simulink model "Modell_13_1"  (R2018a)
settings: Solver=VariableStepAuto  StartTime=0.0  StopTime=10.0  RelTol=1e-3
InitFcn:
  | init_13_1
values from neighbouring files (symbols this model uses):
  b = 1    [init_13_1.m]    (also in init_13_3.m)
  c = 1    [init_13_1.m]    (also in init_13_3.m)
settings Model: Creator=Uni  LastModifiedBy=Uni

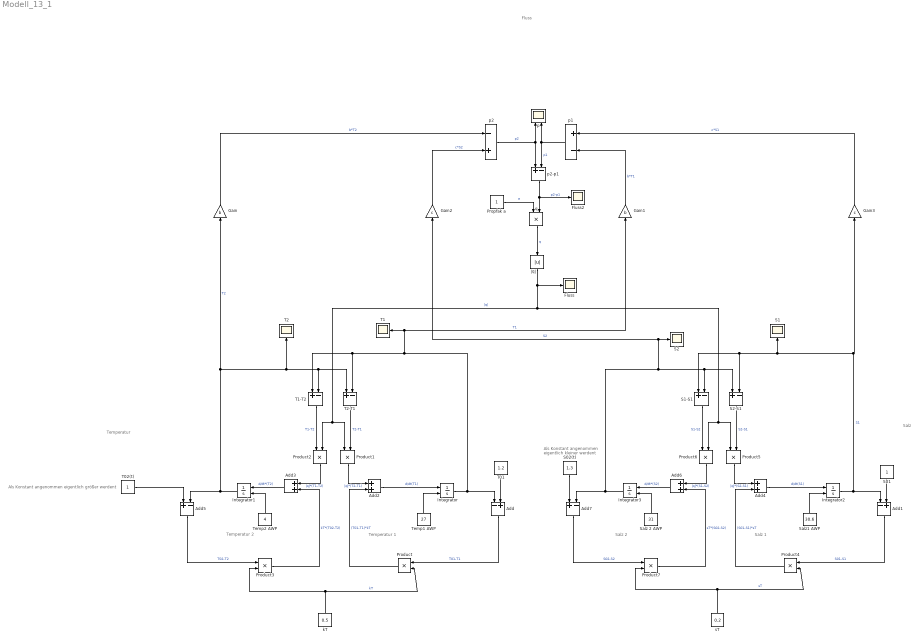
== system Modell_13_1 ==
  note: Als Konstant angenommen eigentlich größer werdent
  note: Temperatur 1
  note: Temperatur 2
  note: Als Konstant angenommen
      | eigentlich kleiner werdent
  note: Salz 2
  note: Salz 1
  note: Temperatur
  note: Salz
  note: Fluss
  Add : Sum  Inputs=-+
  Add1 : Sum  Inputs=-+
  Add{2..4,6} (4 alike) : Sum
  Add5 : Sum  Inputs=+-
  Add7 : Sum  Inputs=+-
  Fluss : Scope
  Fluss2 : Scope
  Gain : Gain  Gain=b
  Gain1 : Gain  Gain=b
  Gain2 : Gain  Gain=c
  Gain3 : Gain  Gain=c
  Integrator{,1..3} (4 alike) : Integrator  InitialConditionSource=external
  Product{,1..7} (8 alike) : Product
  Propfak a : Constant
  S01 : Constant
  S02(t) : Constant  Value=1.3
  S1 : Scope
  S1-S1 : Sum  Inputs=+-
  S2 : Scope
  S2-S1 : Sum  Inputs=+-
  Salz 2 AWP : Constant  Value=31
  Salz1 AWP : Constant  Value=30.6
  T01 : Constant  Value=1.2
  T02(t) : Constant
  T1 : Scope
  T1-T2 : Sum  Inputs=+-
  T2 : Scope
  T2-T1 : Sum  Inputs=+-
  Temp1 AWP : Constant  Value=27
  Temp2 AWP : Constant  Value=4
  kT : Constant  Value=0.5
  p : Scope  NumInputPorts=2
  p1 : Sum  Inputs=+-
  p2 : Sum  Inputs=-+
  p2-p1 : Sum  Inputs=+-
  q : Product
  sT : Constant  Value=0.2
  |q| : Abs
  wires:
  Add2/1 -> Integrator/1  "d/dt(T1)"
  Integrator/1 -> Add/1, T2-T1/2, T1-T2/1, Gain1/1, T1/1  "T1"
  Add/1 -> Product/1  "T01-T1"
  Temp1 AWP/1 -> Integrator/2
  kT/1 -> Product/2, Product3/2  "kT"
  Product/1 -> Add2/2  "(T01-T1)*kT"
  T2-T1/1 -> Product1/2  "T2-T1"
  Product1/1 -> Add2/1  "|q|*(T2-T1)"
  Product2/1 -> Add3/1  "|q|*(T1-T2)"
  T1-T2/1 -> Product2/1  "T1-T2"
  Add3/1 -> Integrator1/1  "d/dt*(T2)"
  Temp2 AWP/1 -> Integrator1/2
  Integrator1/1 -> Add5/2, T2/1, T1-T2/2, T2-T1/1, Gain/1  "T2"
  Product3/1 -> Add3/2  "kT*(T02-T2)"
  Add5/1 -> Product3/1  "T02-T2"
  T01/1 -> Add/2
  Add4/1 -> Integrator2/1  "d/dt(S1)"
  Product4/1 -> Add4/2  "(S01-S1)*sT"
  Add7/1 -> Product7/1  "S02-S2"
  sT/1 -> Product4/2, Product7/2  "sT"
  Salz1 AWP/1 -> Integrator2/2
  Add1/1 -> Product4/1  "S01-S1"
  Product6/1 -> Add6/1  "|q|*(S1-S2)"
  |q|/1 -> Fluss/1, Product5/1, Product6/2, Product1/1, Product2/2  "|q|"
  S2-S1/1 -> Product5/2  "S2-S1"
  Salz 2 AWP/1 -> Integrator3/2
  Add6/1 -> Integrator3/1  "d/dt*(S2)"
  Product7/1 -> Add6/2  "sT*(S02-S2)"
  Integrator2/1 -> Add1/1, Gain3/1, S2-S1/2, S1-S1/1, S1/1  "S1"
  S01/1 -> Add1/2
  Integrator3/1 -> Add7/2, S1-S1/2, S2-S1/1, Gain2/1, S2/1  "S2"
  Product5/1 -> Add4/1  "|q|*(S2-S1)"
  S1-S1/1 -> Product6/1  "S1-S2"
  q/1 -> |q|/1  "q"
  Propfak a/1 -> q/1  "a"
  p2-p1/1 -> q/2, Fluss2/1  "p2-p1"
  p1/1 -> p/2, p2-p1/2  "p1"
  p2/1 -> p/1, p2-p1/1  "p2"
  Gain/1 -> p2/1  "b*T2"
  Gain1/1 -> p1/2  "b*T1"
  Gain2/1 -> p2/2  "c*S2"
  Gain3/1 -> p1/1  "c*S1"
  T02(t)/1 -> Add5/1
  S02(t)/1 -> Add7/1
